simulink model "closed_loop"  (R2023b)
settings: Solver=VariableStepAuto  StartTime=0.0  StopTime=6  RelTol=1e-3
settings Model: Creator=david.wong  LastModifiedBy=david.wong

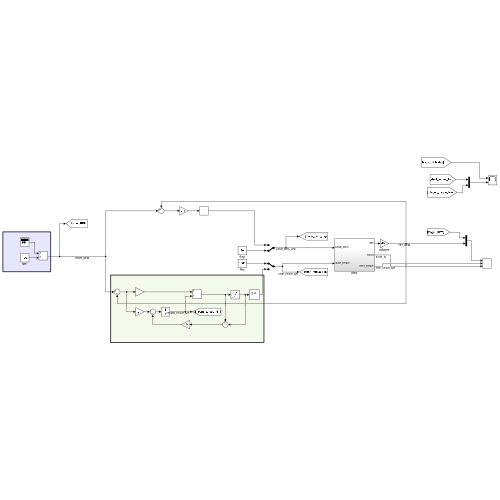
[thumbnail: Simulink's stored preview of the top-level diagram]
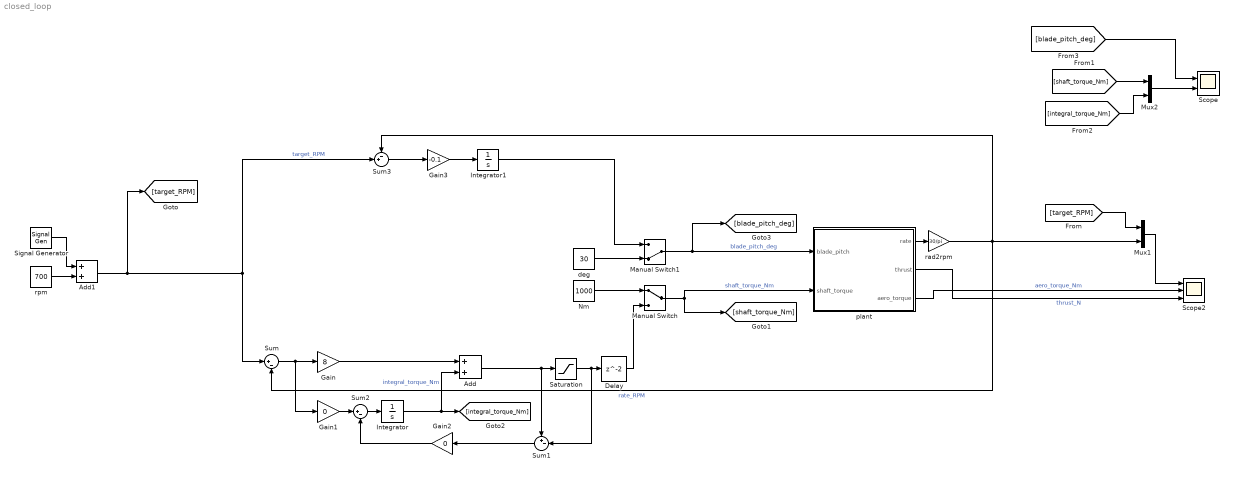
== system closed_loop ==
  Add : Sum
  Add1 : Sum
  Delay : Delay  SampleTime=0.01
  Gain : Gain  Gain=8
  Gain1 : Gain  Gain=0
  Gain2 : Gain  Gain=0
  Gain3 : Gain  Gain=-0.1
  Integrator : Integrator
  Integrator1 : Integrator  InitialCondition=30
  Manual Switch : ManualSwitch
  Manual Switch1 : ManualSwitch  CurrentSetting=0
  Mux1 : Mux  Inputs=2
  Mux2 : Mux  Inputs=2
  Nm : Constant  Value=1000
  Saturation : Saturate  UpperLimit=2000  LowerLimit=-1000
  Scope : Scope  NumInputPorts=2
  Scope2 : Scope  NumInputPorts=3
  Signal Generator : SignalGenerator  WaveForm=square  Amplitude=100  Frequency=0.25
  Sum : Sum  Inputs=|+-
  Sum1 : Sum  Inputs=+-|
  Sum2 : Sum  Inputs=|+-
  Sum3 : Sum  Inputs=-+|
  deg : Constant  Value=30
  plant : Subsystem
  rad2rpm : Gain  Gain=30/pi
  rpm : Constant  Value=700
  wires:
  Manual Switch/1 -> [shaft_torque_Nm], plant/2(shaft_torque)  "shaft_torque_Nm"
  Manual Switch1/1 -> [blade_pitch_deg], plant/1(blade_pitch)  "blade_pitch_deg"
  plant/1(rate) -> rad2rpm/1
  rad2rpm/1 -> Mux1/2, Sum3/1, Sum/2  "rate_RPM"
  Nm/1 -> Manual Switch/1
  deg/1 -> Manual Switch1/2
  Add1/1 -> [target_RPM], Sum3/2, Sum/1  "target_RPM"
  Sum/1 -> Gain1/1, Gain/1
  Gain/1 -> Add/1
  Delay/1 -> Manual Switch/2
  Saturation/1 -> Delay/1, Sum1/2
  Integrator/1 -> [integral_torque_Nm], Add/2  "integral_torque_Nm"
  Add/1 -> Saturation/1, Sum1/1
  rpm/1 -> Add1/2
  Signal Generator/1 -> Add1/1
  Sum1/1 -> Gain2/1
  Gain1/1 -> Sum2/1
  Sum2/1 -> Integrator/1
  Gain2/1 -> Sum2/2
  Sum3/1 -> Gain3/1
  Gain3/1 -> Integrator1/1
  Integrator1/1 -> Manual Switch1/1
  Mux1/1 -> Scope2/1
  [target_RPM] -> Mux1/1
  [integral_torque_Nm] -> Mux2/2
  plant/3(aero_torque) -> Scope2/2  "aero_torque_Nm"
  plant/2(thrust) -> Scope2/3  "thrust_N"
  [shaft_torque_Nm] -> Mux2/1
  Mux2/1 -> Scope/2
  [blade_pitch_deg] -> Scope/1

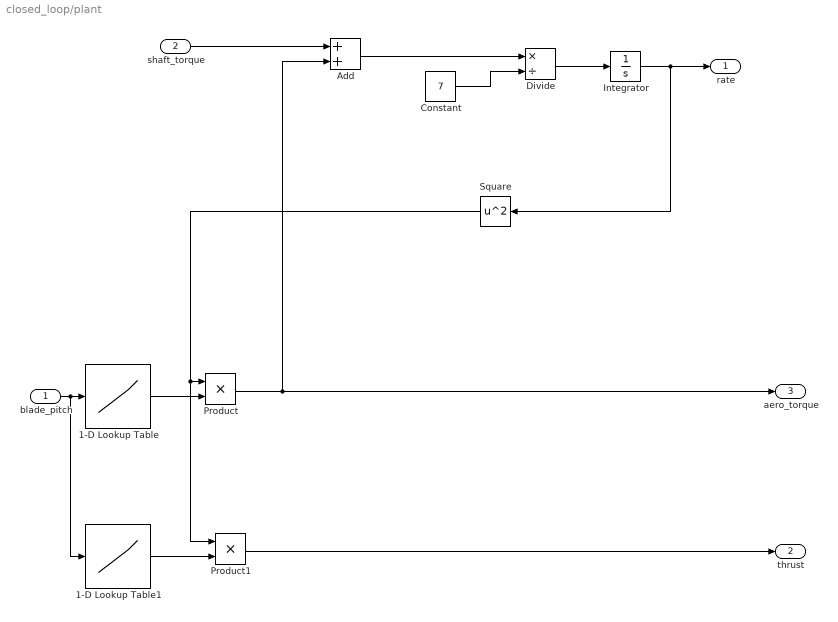
== system closed_loop/plant ==
  blade_pitch : Inport
  shaft_torque : Inport  Port=2
  1-D Lookup Table : Lookup_n-D  NumberOfTableDimensions=1  BreakpointsForDimension1=[0 10 20 30 40 50 60]  Table=[-0.1 0.1 0 -0.1 -0.2 -0.4 -0.8]  InternalRulePriority=Speed  RndMeth=Simplest
  1-D Lookup Table1 : Lookup_n-D  NumberOfTableDimensions=1  BreakpointsForDimension1=[0 10 20 30 40 50 60]  Table=[-1 -0.5 0 0.5 1 0.9 0.8]  InternalRulePriority=Speed  RndMeth=Simplest
  Add : Sum
  Constant : Constant  Value=7
  Divide : Product  Inputs=*/
  Integrator : Integrator
  Product : Product
  Product1 : Product
  Square : Math  Operator=square
  rate : Outport
  thrust : Outport  Port=2
  aero_torque : Outport  Port=3
  wires:
  Constant/1 -> Divide/2
  Divide/1 -> Integrator/1
  Integrator/1 -> Square/1, rate/1
  Add/1 -> Divide/1
  blade_pitch/1 -> 1-D Lookup Table1/1, 1-D Lookup Table/1
  shaft_torque/1 -> Add/1
  1-D Lookup Table/1 -> Product/2
  Square/1 -> Product1/1, Product/1
  1-D Lookup Table1/1 -> Product1/2
  Product1/1 -> thrust/1
  Product/1 -> aero_torque/1, Add/2
